simulink model "LuGre_model"  (R2026a)
settings: Solver=VariableStepAuto
settings Model: Creator=shuki  LastModifiedBy=shuki

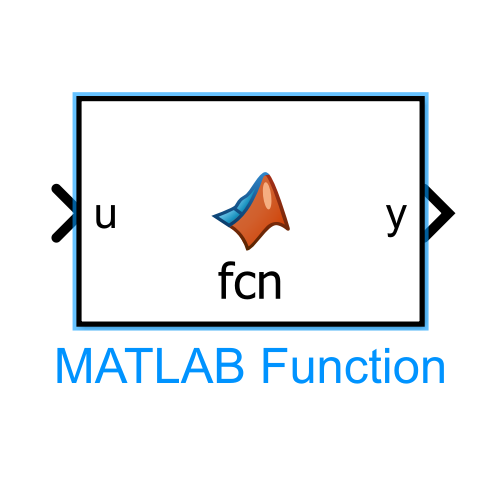
[thumbnail: Simulink's stored preview of the top-level diagram]
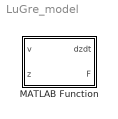
== system LuGre_model ==
  MATLAB Function : MATLAB Function  TreatAsAtomicUnit=on

== matlab function LuGre_model/MATLAB Function ==
  data: v input; dzdt output; z input; F output
function [dzdt, F] = lugre_model(v, z)
% parameters (from the table I in the paper of LuGre) 
sigma0 = 1e5; % stiffness, refined
sigma1 = sqrt(sigma0); % damping(減衰)
sigma2 = 0.4; % viscosity coefficient(粘性係数)
Fc = 1.0; % dynamic friction force(動摩擦力)
Fs = 1.5; % static friction force(静止摩擦力)
vs = 0.001; % stribeck speed(ストライベック速度)

% g(v)
gv = Fc + (Fs - Fc) * exp(-(v/vs)^2);

% dz/dt
dzdt = v - (sigma0 * abs(v) / gv) * z;

% F
F = sigma0 * z + sigma1 * dzdt + sigma2 * v;
end
